simulink model "rtwdemo_buildinfo"  (Simulink 7.6)
settings: Solver=FixedStepDiscrete  StartTime=0.0  StopTime=10.0  FixedStep=0.01  RelTol=1e-3
PreLoadFcn:
  | addpath(fullfile(matlabroot,'toolbox','rtw','rtwdemos','buildinfo_demo'));
libraries: rtwdemowidgets x1
Description:
  | Exporting Generated Files Using PackNGo and BuildInfo API
CloseFcn:
  | rmpath(fullfile(matlabroot,'toolbox','rtw','rtwdemos','buildinfo_demo'));
settings Model: Creator=The MathWorks Inc.  ExtModeAutoUpdateStatusClock=off
settings MATStruct: SampleTime=0.01  Offset=0  Priority=[20.0]
settings DataIOCC: SaveOutput=off  SaveTime=off
settings OptimizationCC: InlineParams=on  InlineInvariantSignals=on  StateBitsets=on  DataBitsets=on  UseTempVars=on  EfficientFloat2IntCast=on  EfficientMapNaN2IntZero=off
settings DebuggingCC: SolverPrmCheckMsg=none  StrictBusMsg=ErrorOnBusTreatedAsVector
settings HardwareCC: ProdIntDivRoundTo=Zero  ProdEndianess=LittleEndian  ProdHWDeviceType=Generic->32-bit Embedded Processor  TargetHWDeviceType=Generic->32-bit Embedded Processor
settings RTWCC: PostCodeGenCommand=rtwdemo_buildinfo_data(buildInfo)  GenerateReport=on  RTWVerbose=off  ProcessScript=grt_make_rtw_hook  CustomInclude=buildinfo_demo  CustomSource=buildinfo_custom_src.c  LaunchReport=on  IncludeERTFirstTime=on
settings CodeAppCC: ForceParamTrailComments=on
settings GRTTargetCC: TargetFcnLib=ansi_tfl_tmw.mat

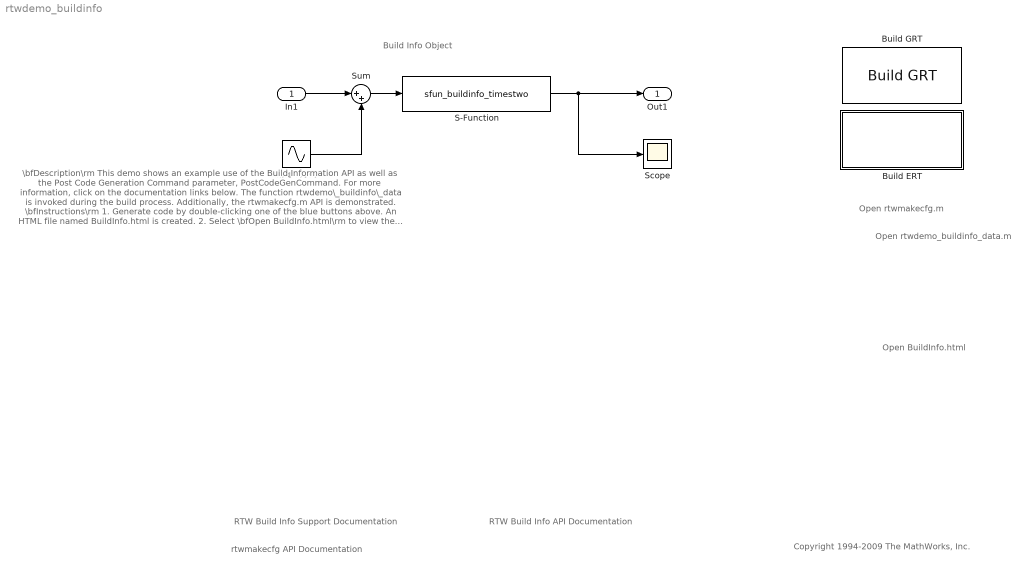
== system rtwdemo_buildinfo ==
  note: Build Info Object
  note: \bfDescription\rm
      |  This demo shows an example use of the Build Information API as well as the Post Code Generation
      |  Command parameter, PostCodeGenCommand.  For more information, click on the documentation
      |  links below.
      |  The function rtwdemo\_buildinfo\_data is invoked during the build process.  Additionally, the
      |  rtwmakecfg.m API is demonstrated.
      |
      | \bfInstructions\rm
      | 1. Generate code by double-clicking one of the blue buttons above. An HTML file named
      |     BuildInfo.html is created.
      | 2. Select \bfOpen BuildInfo.html\rm to view the file in a Web browser. Follow the hyperlinks to
      |     open the source files listed.
      |
      | \bfNotes\rm
      | 1. Use \bfget\_param('rtwdemo\_buildinfo', 'PostCodeGenCommand')\rm to see the function
      |     executed in the Post Code Gen Command stage.
      | 2. Select \bfOpen rtwdemo\_buildinfo\_data.m\rm to study the API for the Build Info object.
      | 3. Select \bfOpen rtwmakecfg.m\rm to study the use of rtwmakecfg API.
      | 4. The buildInfo object is saved out to the following location  \bfrtwdemo\_<target>\_rtw\\buildInfo.mat\rm
      | 5. The \bfpackNGo\rm feature of the buildInfo object is invoked at the end of the post code generation
      |     function \bfrtwdemo\_buildinfo\_data.m
  note: Open rtwdemo_buildinfo_data.m
  note: Open BuildInfo.html
  note: RTW Build Info Support Documentation
  note: RTW Build Info API Documentation
  note: rtwmakecfg API Documentation
  note: Open rtwmakecfg.m
  note: Copyright 1994-2009 The MathWorks, Inc.
  In1 : Inport  OutDataTypeStr=double  PortDimensions=1  SampleTime=0.01
  Build ERT : Subsystem  mask{attrib_overrides={'IncludeMdlTerminateFcn', 'ERTFilePackagingFormat'}}
      mask prompts: attrib_overrides "List of attributes to preserve (cell of strings):"
      mask help: Enter the attributes of the configuration set that you want preserved. Otherwise, the default configuration script will override your current settings.
      settings: OpenFcn=|
      | model=bdroot;                                                       overrides=get_param(gcb,'attrib_overrides');
      | 
      | try   rtwconfiguredemo(model,'noop',false,overrides);
      | set_param(model,'SupportContinuousTime','on');
      | set_param(model,'SupportNonInlinedSFcns','on');
      |   set_param(model,'SupportNonFinite','on');
      |   set_param(model,'SupportComplex','on');     % set_param(model,'GenerateReport','off');
      |    rtwbuilddemomodel(model);
      | catch
      |    error(lasterr);
      | end
      |                                       clear model overrides;
      mask Display:
      | disp(['Generate Code Using\n',...
      | 	  'Real-Time Workshop\n',...
      | 	  'Embedded Coder\n'...
      | 	  '(double-click)'])
  Build GRT : rtwdemowidgets/Build GRT  SystemSampleTime=-1  attrib_overrides={}
  S-Function : S-Function  FunctionName=sfun_buildinfo_timestwo  SFunctionModules='sfun_buildinfo_src_module'  EnableBusSupport=off
  Scope : Scope
  Sine Wave : Sin  Amplitude=2  SampleTime=0
  Sum : Sum  Inputs=|++
  Out1 : Outport
  wires:
  S-Function/1 -> Scope/1, Out1/1
  In1/1 -> Sum/1
  Sine Wave/1 -> Sum/2
  Sum/1 -> S-Function/1

== system rtwdemo_buildinfo/Build ERT ==
